simulink subsystem "baro_lut_controller"  (R2024b)
settings: Solver=VariableStepAuto  StartTime=0.0  StopTime=10.0  RelTol=1e-3
undefined symbols (not defined in the file or in its folder): baro_lut, const_brake, controller_rate, dspblkCoreblockFVToolHelper, gcbh, pos_den, pos_num, position_init, vel_den, vel_num, velocity_init
libraries: simulink x1
settings Model: Creator=yevge  LastModifiedBy=yevge

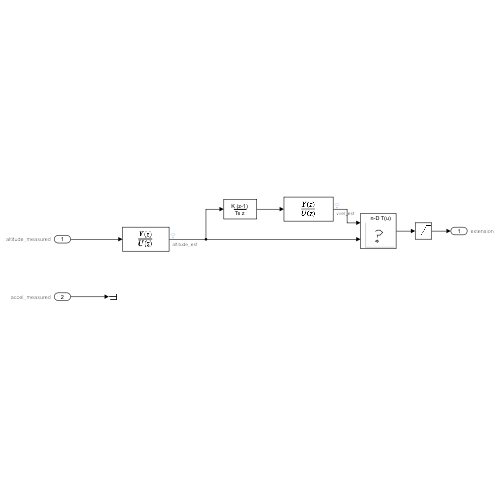
[thumbnail: Simulink's stored preview of the top-level diagram]
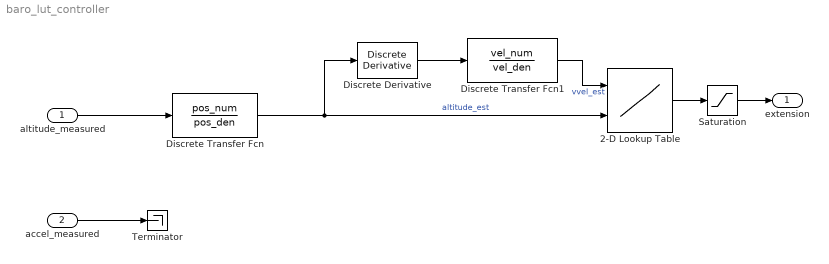
== system baro_lut_controller ==
  altitude_measured : Inport  Unit=m  PortDimensions=1  SampleTime=1/controller_rate
  accel_measured : Inport  Port=2  Unit=m/s^2  PortDimensions=[2 1]  SampleTime=1/controller_rate
  2-D Lookup Table : Lookup_n-D  BreakpointsForDimension1=baro_lut.vel  BreakpointsForDimension2=baro_lut.alt  Table=baro_lut{:, :}  InternalRulePriority=Speed  RndMeth=Simplest
      settings: InputPortMap=u0,u1
  Discrete Transfer Fcn : DiscreteTransferFcn  LoadFcn=dspblkCoreblockFVToolHelper(gcbh,'load');  Numerator=pos_num  Denominator=pos_den  InitialStates=position_init(2)  a0EqualsOne=on
      settings: CopyFcn=dspblkCoreblockFVToolHelper(gcbh,'copy');  DeleteFcn=dspblkCoreblockFVToolHelper(gcbh,'close');  ModelCloseFcn=dspblkCoreblockFVToolHelper(gcbh,'close');  PreSaveFcn=dspblkCoreblockFVToolHelper(gcbh,'presave');  PostSaveFcn=dspblkCoreblockFVToolHelper(gcbh,'postsave');  CloseFcn=dspblkCoreblockFVToolHelper(gcbh,'close');
  Discrete Transfer Fcn1 : DiscreteTransferFcn  LoadFcn=dspblkCoreblockFVToolHelper(gcbh,'load');  Numerator=vel_num  Denominator=vel_den  InitialStates=velocity_init(2)  a0EqualsOne=on
      settings: CopyFcn=dspblkCoreblockFVToolHelper(gcbh,'copy');  DeleteFcn=dspblkCoreblockFVToolHelper(gcbh,'close');  ModelCloseFcn=dspblkCoreblockFVToolHelper(gcbh,'close');  PreSaveFcn=dspblkCoreblockFVToolHelper(gcbh,'presave');  PostSaveFcn=dspblkCoreblockFVToolHelper(gcbh,'postsave');  CloseFcn=dspblkCoreblockFVToolHelper(gcbh,'close');
  Discrete Derivative : simulink/Discrete/Discrete Derivative  gainval=1.0  ICPrevScaledInput=0.0  OutMin=[]  OutMax=[]  OutDataType=fixdt(1, 16)  OutScaling=2^-10  DoSatur=off
  Saturation : Saturate  UpperLimit=1  LowerLimit=0
  Terminator : Terminator
  extension : Outport  OutMin=0  OutMax=1  Unit=1  PortDimensions=1  SampleTime=1/controller_rate  InitialOutput=const_brake
  wires:
  accel_measured/1 -> Terminator/1
  altitude_measured/1 -> Discrete Transfer Fcn/1
  Discrete Transfer Fcn/1 -> 2-D Lookup Table/2, Discrete Derivative/1  "altitude_est"
  2-D Lookup Table/1 -> Saturation/1
  Discrete Derivative/1 -> Discrete Transfer Fcn1/1
  Discrete Transfer Fcn1/1 -> 2-D Lookup Table/1  "vvel_est"
  Saturation/1 -> extension/1
